simulink model "setpointToOutput_th"  (R2018b)
settings: Solver=VariableStepAuto  StartTime=0.0  StopTime=10.0  RelTol=1e-3
values from neighbouring files (symbols this model uses):
  chi_des = 10*pi/180    (= 0.174532925199)    [setpointToOutput_ts.m]
  eul_ang = [0;45*pi/180;0;]    [setpointToOutput_ts.m]
  flow = [1;0;0;]    [setpointToOutput_ts.m]    (also in testUntilRoll_ts.m)
  pos = [1;0;1;]    [setpointToOutput_ts.m]
  vel = [-1;0;1;]    [setpointToOutput_ts.m]
libraries: setpointToOutput_cl x1
settings Model: Creator=jldanie5  LastModifiedBy=jldanie5

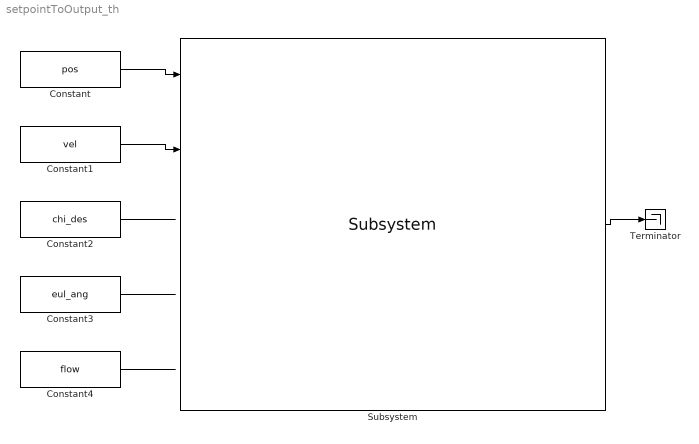
== system setpointToOutput_th ==
  Constant : Constant  Value=pos
  Constant1 : Constant  Value=vel
  Constant2 : Constant  Value=chi_des
  Constant3 : Constant  Value=eul_ang
  Constant4 : Constant  Value=flow
  Subsystem : setpointToOutput_cl/Subsystem  AoA_des=0  controlMat=0  ctrlSigMax=0
  Terminator : Terminator
  wires:
  Constant/1 -> Subsystem/1
  Constant1/1 -> Subsystem/2
  Constant2/1 -> ?
  Constant3/1 -> ?
  Constant4/1 -> ?
  Subsystem/1 -> Terminator/1
